simulink model "Three_Input_Model_Output"  (R2021a)
settings: Solver=VariableStepAuto  StartTime=0.0  StopTime=10.0  RelTol=1e-3
values from neighbouring files (symbols this model uses):
  A = double(subs(a,[x;u],equil))    [Funwork3_Main.m]    (also in Values.mat = [0 0 0 0 0 0 0 0 0 -8.175 65.4 -32.7 ... (36 elements, 6x6)]; Values_Rev2.mat = [0 0 0 0 0 0 0 0 0 -8.175 65.4 -32.7 ... (36 elements, 6x6)]; Values_Rev3.mat = [0 0 0 0 0 0 0 0 0 -0.534142885228 22.5045950602 -13.9882516)
  B = double(subs(b,[x;u],equil))    [Funwork3_Main.m]    (also in Values.mat = [0 0 0 0.666666666667 -1.33333333333 0]; Values_Rev2.mat = [0  0; 0  0; 0  0; 0.666666666667  -1.33333333333; -1.333333; Values_Rev3.mat = [0 0 0 0.425188099574 -0.174236211288 -0.288671680413 0 0 0 )
  C = [1 0 0 0 0 0 ... (first row only)    [Funwork3_Main.m]    (also in Values.mat = [1 0 0 0 1 0 0 0 1 0 0 0 ... (18 elements, 3x6)]; Values_Rev2.mat = [1 0 0 0 1 0 0 0 1 0 0 0 ... (18 elements, 3x6)]; Values_Rev3.mat = [1 0 0 0 1 0 0 0 1 0 0 0 ... (18 elements, 3x6)])
  D = zeros(3,3)    [Funwork3_Main.m]    (also in Values.mat = [0 0 0]; Values_Rev2.mat = [0  0; 0  0; 0  0]; Values_Rev3.mat = [0  0  0; 0  0  0; 0  0  0])
  K = M^-1*N    [Funwork3_Main.m]    (also in Values_Rev2.mat = [-2.68055786937  1.11424421179  -57.4156910728  -4.790622744; Values_Rev3.mat = [1104.07953515 279.420010905 157.104315976 182.686027553 129)
  u_e = zeros(3,1)    [Funwork3_Main.m]    (also in Values_Rev3.mat = [0 9.21172186389 3.90190360694])
  x0 = [0;-50*pi/180;-40*pi/180;0;0;0]    [Funwork3_Main.m]
  x_e = [0.1;theta1;theta2;0;0;0]    [Funwork3_Main.m]    (also in Values_Rev3.mat = [0.1 -1.0471975512 -0.785398163397 0 0 0])
undefined symbols (not defined in the file or in its folder): v
libraries: vrlib x2, aerolibanimutils x1, dspvision x1
settings Model: Creator=J44381  LastModifiedBy=vicen
settings SolverCC: AlgebraicLoopSolver=TrustRegion
settings DebuggingCC: SFMachineParentedDataDiag=warning

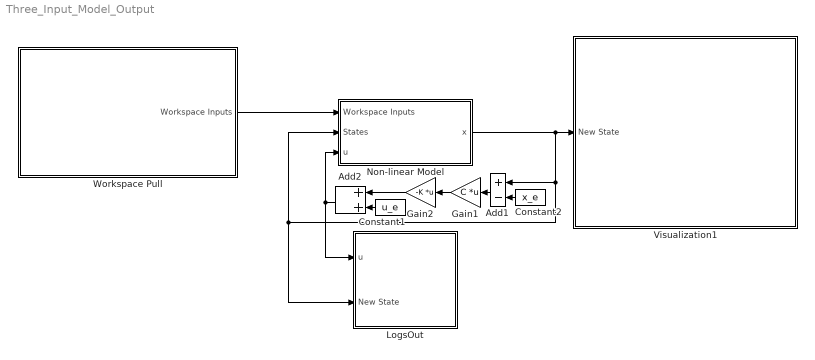
== system Three_Input_Model_Output ==
  Add1 : Sum  Inputs=+-
  Add2 : Sum
  Constant1 : Constant  Value=u_e
  Constant2 : Constant  Value=x_e
  Gain1 : Gain  Gain=C  Multiplication=Matrix(K*u)
  Gain2 : Gain  Gain=-K  Multiplication=Matrix(K*u)
  LogsOut : Subsystem
  Non-linear Model : Subsystem
  Visualization1 : Subsystem
  Workspace Pull : Subsystem
  wires:
  Workspace Pull/1("Workspace Inputs ") -> Non-linear Model/1("Workspace Inputs ")
  Add2/1 -> LogsOut/1(u), Non-linear Model/3(u)
  Gain2/1 -> Add2/1
  Constant1/1 -> Add2/2
  Constant2/1 -> Add1/2
  Add1/1 -> Gain1/1
  Non-linear Model/1(x) -> Visualization1/1(New State), LogsOut/2(New State), Non-linear Model/2(States), Add1/1
  Gain1/1 -> Gain2/1

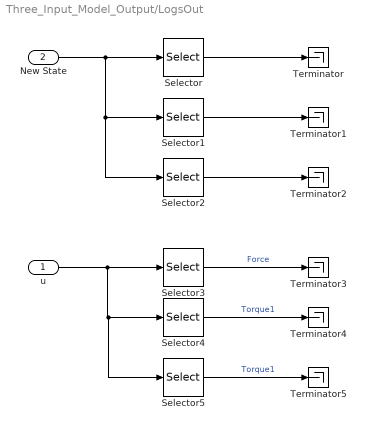
== system Three_Input_Model_Output/LogsOut ==
  u : Inport
  New State : Inport  Port=2
  Selector : Selector  InputPortWidth=6  IndexOptions=Index vector (dialog)  Indices=1  OutputSizes=1
  Selector1 : Selector  InputPortWidth=6  IndexOptions=Index vector (dialog)  Indices=2  OutputSizes=1
  Selector2 : Selector  InputPortWidth=6  IndexOptions=Index vector (dialog)  Indices=3  OutputSizes=1
  Selector3 : Selector  InputPortWidth=3  IndexOptions=Index vector (dialog)  Indices=1  OutputSizes=1
  Selector4 : Selector  InputPortWidth=3  IndexOptions=Index vector (dialog)  Indices=2  OutputSizes=1
  Selector5 : Selector  InputPortWidth=3  IndexOptions=Index vector (dialog)  Indices=3  OutputSizes=1
  Terminator{,1..5} (6 alike) : Terminator
  wires:
  Selector/1 -> Terminator/1
  Selector1/1 -> Terminator1/1
  Selector2/1 -> Terminator2/1
  New State/1 -> Selector2/1, Selector1/1, Selector/1
  u/1 -> Selector5/1, Selector4/1, Selector3/1
  Selector4/1 -> Terminator4/1  "Torque1"
  Selector3/1 -> Terminator3/1  "Force"
  Selector5/1 -> Terminator5/1  "Torque1"

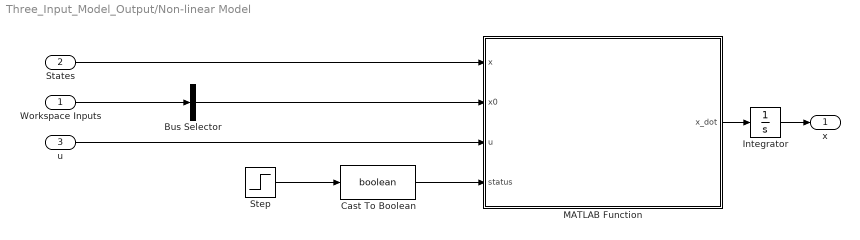
== system Three_Input_Model_Output/Non-linear Model ==
  "Workspace Inputs " : Inport
  States : Inport  Port=2
  u : Inport  Port=3
  Bus Selector : BusSelector  OutputSignals=Initial_States  OutputAsBus=on
  Cast To Boolean : DataTypeConversion  OutDataTypeStr=boolean
  Integrator : Integrator  InitialCondition=[x0.x;x0.theta1;x0.theta2;x0.x_dot;x0.theta1_dot;x0.theta2_dot]
  MATLAB Function : MATLAB Function  TreatAsAtomicUnit=on
  Step : Step  Time=.01  SampleTime=0
  x : Outport
  wires:
  MATLAB Function/1(x_dot) -> Integrator/1
  States/1 -> MATLAB Function/1(x)
  "Workspace Inputs "/1 -> Bus Selector/1
  u/1 -> MATLAB Function/3(u)
  Bus Selector/1 -> MATLAB Function/2(x0)
  Step/1 -> Cast To Boolean/1
  Cast To Boolean/1 -> MATLAB Function/4(status)
  Integrator/1 -> x/1

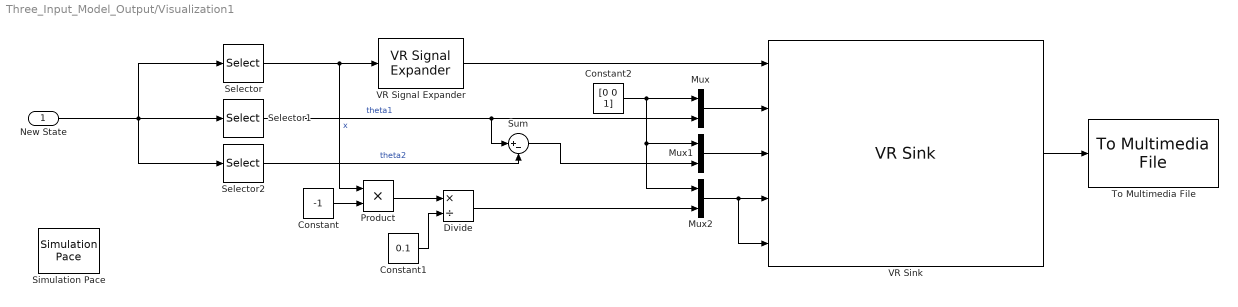
== system Three_Input_Model_Output/Visualization1 ==
  New State : Inport
  Constant : Constant  Value=-1
  Constant1 : Constant  Value=0.1
  Constant2 : Constant  Value=[0 0 1]
  Divide : Product  Inputs=*/
  Mux : Mux  Inputs=2
  Mux1 : Mux  Inputs=2
  Mux2 : Mux  Inputs=2
  Product : Product
  Selector : Selector  InputPortWidth=6  IndexOptions=Index vector (dialog)  Indices=1  OutputSizes=1
  Selector1 : Selector  InputPortWidth=6  IndexOptions=Index vector (dialog)  Indices=2  OutputSizes=1
  Selector2 : Selector  InputPortWidth=6  IndexOptions=Index vector (dialog)  Indices=3  OutputSizes=1
  Simulation Pace : aerolibanimutils/Simulation Pace  SimulationPace=1  SleepMode=Auto  OutputPaceError=off  SampleTime=1/30
  Sum : Sum  Inputs=|+-
  To Multimedia File : dspvision/To Multimedia File  outputFilename=output.avi  streamSelection=Video only  videoCompressor=None (uncompressed)  audioCompressor=None (uncompressed)  imagePorts=One multidimensional signal  fileType=AVI  audioDatatype=Determine from input data type  fourcc=RGB  videoQuality=75  mj2000CompFactor=10
  VR Signal Expander : vrlib/VR Signal Expander  outwidth=3  outidx=[1]
  VR Sink : vrlib/VR Sink  InstantiateOnLoad=on  SampleTime=0.1  ViewEnable=on  RemoteChange=off  RemoteView=off  FieldsWritten=Cart.translation.3.1.1.double#Rotation1.rotation.4.1.1.double#Rotation2.rotation.4.1.1.double#Axis_Rotate.rotation.4.1.1.double#Axis_Rotate2.rotation.4.1.1.double  WorldFileName=Cart_Actual.WRL  AutoView=off  VideoDimensions=[1500 2000]  AllowVariableSize=off  FigureProperties="{'Position', 'Name', 'Viewpoint', 'CameraBound', 'CameraDirection', 'CameraPosition', 'CameraUpVector', 'ZoomFactor', 'Antialiasing', 'Headlight', 'Lighting', 'NavPanel', 'Sound', 'StatusBar', 'Stereo3D', 'Stereo3DCameraOffset', 'Stereo3DHIT', 'ToolBar', 'Textures', 'Transparency', 'Triad', 'Wireframe', 'NavZones', 'NavMode', 'NavSpeed', 'CaptureFileFormat', 'CaptureFileName', 'Record2DCompressMethod', 'Record2DCompressQuality', 'Record2D', 'Record2DFileName', 'Record2DFPS'; [1.2660000000000001e+02   9.4799999999999955e+01   8.0000000000000000e+02   6.0020000000000005e+02], '', '_untitled_1', 'on', [0.0000000000000000e+00   0.0000000000000000e+00  -1.0000000000000000e+00], [0.0000000000000000e+00   0.0000000000000000e+00   0.0000000000000000e+00], [0.0000000000000000e+00   1.0000000000000000e+00   0.0000000000000000e+00], [1.0000000000000000e+00], 'on', 'on', 'on', 'none', 'on', 'off', 'off', [1.0000000149011612e-01], [0.0000000000000000e+00], 'off', 'on', 'on', 'none', 'off', 'off', 'fly', 'normal', 'tif', '%f_anim_%n.tif', 'auto', [7.5000000000000000e+01], 'off', '***video***', 'auto'}"
  wires:
  New State/1 -> Selector/1, Selector2/1, Selector1/1
  Selector/1 -> VR Signal Expander/1, Product/1  "x"
  Selector1/1 -> Sum/1, Mux/2  "theta1"
  Product/1 -> Divide/1
  Constant/1 -> Product/2
  Constant1/1 -> Divide/2
  Constant2/1 -> Mux1/1, Mux2/1, Mux/1
  Selector2/1 -> Sum/2  "theta2"
  Divide/1 -> Mux2/2
  Sum/1 -> Mux1/2
  VR Signal Expander/1 -> VR Sink/1
  Mux/1 -> VR Sink/2
  Mux1/1 -> VR Sink/3
  Mux2/1 -> VR Sink/4, VR Sink/5
  VR Sink/1 -> To Multimedia File/1

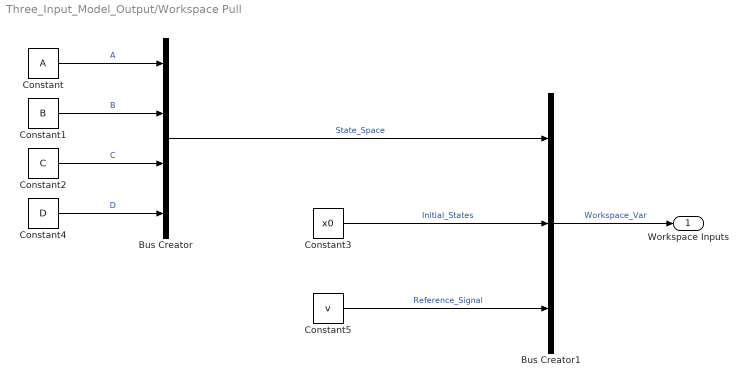
== system Three_Input_Model_Output/Workspace Pull ==
  Bus Creator : BusCreator  Inputs=4
  Bus Creator1 : BusCreator  Inputs=3
  Constant : Constant  Value=A  VectorParams1D=off
  Constant1 : Constant  Value=B  VectorParams1D=off
  Constant2 : Constant  Value=C  VectorParams1D=off
  Constant3 : Constant  Value=x0  VectorParams1D=off  OutDataTypeStr=Bus: State_bus
  Constant4 : Constant  Value=D  VectorParams1D=off
  Constant5 : Constant  Value=v  VectorParams1D=off  OutDataTypeStr=Bus: Reference_bus
  "Workspace Inputs " : Outport
  wires:
  Constant/1 -> Bus Creator/1  "A"
  Constant1/1 -> Bus Creator/2  "B"
  Constant2/1 -> Bus Creator/3  "C"
  Constant4/1 -> Bus Creator/4  "D"
  Bus Creator/1 -> Bus Creator1/1  "State_Space"
  Bus Creator1/1 -> "Workspace Inputs "/1  "Workspace_Var"
  Constant3/1 -> Bus Creator1/2  "Initial_States"
  Constant5/1 -> Bus Creator1/3  "Reference_Signal"

== matlab function Three_Input_Model_Output/Non-linear Model/MATLAB Function ==
  data: x input; x0 input; u input; x_dot output; status input
function x_dot  = Nonlinear_Dynamics(x,x0,u,status)
    if status == false
        x2 = x0.theta1;
        x3 = x0.theta2;
        x4 = x0.x_dot;
        x5 = x0.theta1_dot;
        x6 = x0.theta2_dot;
        u1 = u(1);
        u2 = u(2);
        u3 = u(3);
    else
        x2 = x(2);
        x3 = x(3);
        x4 = x(4);
        x5 = x(5);
        x6 = x(6);
        u1 = u(1);
        u2 = u(2);
        u3 = u(3);
    end
    % Insert Equations
    x_dot = double([
                     x4;
                     x5;
                     x6;
                     -(420*u1 - (2943*sin(2*x2))/2 + 150*x5^2*sin(x2) + (135*x6^2*sin(x3))/2 - 180*u1*cos(2*x2 - 2*x3) + 400*u3*cos(2*x2 - x3) - 840*u2*cos(x2) + 840*u3*cos(x2) - 400*u3*cos(x3) + (135*x6^2*sin(2*x2 - x3))/2 + 360*u2*cos(x2 - 2*x3) - 360*u3*cos(x2 - 2*x3))/(30*(5*cos(2*x2) + 9*cos(2*x2 - 2*x3) - 26));
                     (22800*u3 - 22800*u2 - 26487*sin(x2 - 2*x3) - 91233*sin(x2) + 3600*u2*cos(2*x3) - 3600*u3*cos(2*x3) + 4725*x6^2*sin(x2 - x3) + 750*x5^2*sin(2*x2) - 4000*u3*cos(x2 + x3) + 4200*u1*cos(x2) + 1350*x5^2*sin(2*x2 - 2*x3) - 1800*u1*cos(x2 - 2*x3) + 13600*u3*cos(x2 - x3) + 675*x6^2*sin(x2 + x3))/(150*(5*cos(2*x2) + 9*cos(2*x2 - 2*x3) - 26));
                     -(2700*sin(x2 - x3)*x5^2 + 1215*sin(2*x2 - 2*x3)*x6^2 + 13600*u3 - 26487*sin(2*x2 - x3) + 26487*sin(x3) - 4000*u3*cos(2*x2) + 1800*u1*cos(2*x2 - x3) + 3600*u2*cos(x2 + x3) - 3600*u3*cos(x2 + x3) - 1800*u1*cos(x3) - 12240*u2*cos(x2 - x3) + 12240*u3*cos(x2 - x3))/(135*(5*cos(2*x2) + 9*cos(2*x2 - 2*x3) - 26))
                ]);
            
end
